simulink model "untitled"  (Simulink 7.6)
settings: Solver=ode45  StartTime=0.0  StopTime=0.01  RelTol=1e-3
libraries: simulink x1
settings Model: Creator=Mike  LastModifiedBy=Mike

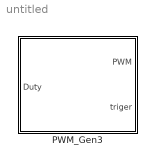
== system untitled ==
  PWM_Gen3 : Subsystem  mask{Ts_Discrete=1e-7, f_tri=10e3, P_Delay=0}
      mask prompts: Ts_Discrete "Sample Time"; f_tri "frequency of sawtooth wave"; P_Delay "Arbittary Phase Delay"

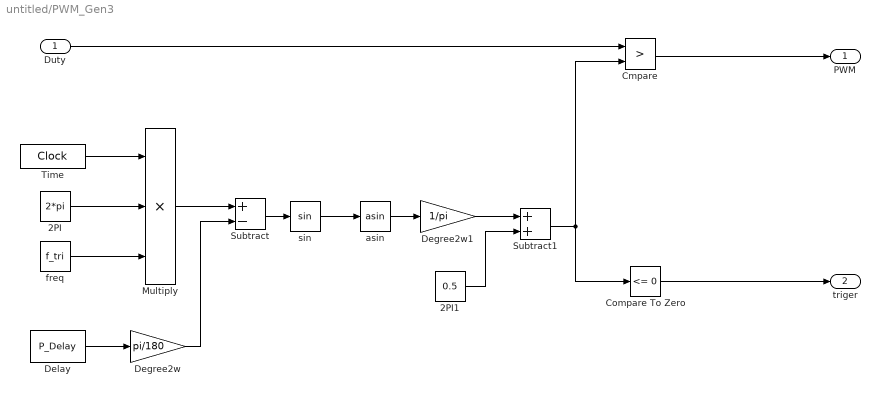
== system untitled/PWM_Gen3 ==
  Duty : Inport
  2PI : Constant  Value=2*pi
  2PI1 : Constant  Value=0.5
  Cmpare : RelationalOperator  Operator=>  OutDataTypeStr=boolean
  Compare To Zero : simulink/Logic and Bit Operations/Compare To Zero  SystemSampleTime=-1  relop=<=  LogicOutDataTypeMode=boolean
  Degree2w : Gain  Gain=pi/180
  Degree2w1 : Gain  Gain=1/pi
  Delay : Constant  Value=P_Delay
  Multiply : Product  Inputs=***
  Subtract : Sum  Inputs=+-
  Subtract1 : Sum
  Time : DigitalClock  SampleTime=Ts_Discrete
  asin : Trigonometry  Operator=asin
  freq : Constant  Value=f_tri
  sin : Trigonometry
  PWM : Outport
  triger : Outport  Port=2
  wires:
  Time/1 -> Multiply/1
  2PI/1 -> Multiply/2
  freq/1 -> Multiply/3
  Multiply/1 -> Subtract/1
  Delay/1 -> Degree2w/1
  Degree2w/1 -> Subtract/2
  Subtract/1 -> sin/1
  sin/1 -> asin/1
  asin/1 -> Degree2w1/1
  Degree2w1/1 -> Subtract1/1
  2PI1/1 -> Subtract1/2
  Subtract1/1 -> Cmpare/2, Compare To Zero/1
  Duty/1 -> Cmpare/1
  Cmpare/1 -> PWM/1
  Compare To Zero/1 -> triger/1
